simulink model "basic_04_sim"  (R2020a)
settings: Solver=FixedStepAuto  StartTime=0.0  StopTime=0.8  FixedStep=0.001  RelTol=1e-3  EnableMultiTasking=on
values from neighbouring files (symbols this model uses):
  m = size(traj)    [testInput.m]
undefined symbols (not defined in the file or in its folder): a1, a2, a3, d1, d4, fc1, fc2, fc3, fc4, fc5, fc6, fv1, fv2, fv3, fv4, fv5, fv6, Ic111, Ic112, Ic113, Ic122, Ic123, Ic133, Ic211, Ic212, Ic213, Ic222, Ic223, Ic233, Ic311, Ic312, Ic313, Ic322, Ic323, Ic333, Ic411, Ic412, Ic413, Ic422, Ic423, Ic433, Ic511, Ic512, Ic513, Ic522, Ic523, Ic533, Ic611, Ic612, Ic613, Ic622, Ic623, Ic633, m1, m2, m3, m4, m5, m6, mc11 ... (+20)
libraries: sm_lib x56, nesl_utility x31
(part 2 of 2)

== matlab function basic_04_sim/ddq6 ==
  data: u input; y output
function y = fcn(u)  
% if u < 0.5    
%     y = -3.14^3*sin(3.14*u);
% else
%     y = -3.14^3*sin(3.14*(1-u));
% end
% y = 10*sin(u);

q0 = 0;
q1 = pi/6;
% q1 = 0;
acc0 = 0;
acc1 = 0; 
t1 = 0.88;
t0 = 0;
v0 = 0;
v1 = 0;

dq = q1-q0;%初始角度差
dt = t1-t0;%时间差

a0 = q0;
a1 = v0;
a2 = acc0/2;
a3 = (20*dq-(8*v1+12*v0)*dt-(3*acc0-acc1)*dt^2)/(2*dt^3);
a4 = (-30*dq+(14*v1+16*v0)*dt+(3*acc0-2*acc1)*dt^2)/(2*dt^4);
a5 = (12*dq-6*(v1+v0)*dt-(acc0-acc1)*dt^2)/(2*dt^5);

y = 2*a2+6*a3*u+12*a4*u.^2+20*a5*u.^3;%角速度

end

== matlab function basic_04_sim/dq6 ==
  data: u input; y output
function y = fcn(u)  
% if u < 0.5    
%     y = 3.14*3.14*cos(3.14*u);
% else
%     y = -3.14*3.14*cos(3.14*(1-u));
% end

q0 = 0;
q1 = pi/6;
% q1 = 0;
acc0 = 0;
acc1 = 0; 
t1 = 0.88;
t0 = 0;
v0 = 0;
v1 = 0;

dq = q1-q0;%初始角度差
dt = t1-t0;%时间差

a0 = q0;
a1 = v0;
a2 = acc0/2;
a3 = (20*dq-(8*v1+12*v0)*dt-(3*acc0-acc1)*dt^2)/(2*dt^3);
a4 = (-30*dq+(14*v1+16*v0)*dt+(3*acc0-2*acc1)*dt^2)/(2*dt^4);
a5 = (12*dq-6*(v1+v0)*dt-(acc0-acc1)*dt^2)/(2*dt^5);

y = a1+2*a2*u+3*a3*u.^2+4*a4*u.^3+5*a5*u.^4;%角速度
end

== matlab function basic_04_sim/q6 ==
  data: u input; y output
function y = fcn(u)  
% if u < 0.5    
%     y = 3.14*sin(3.14*u);
% else
%     y = 3.14*sin(3.14*(1-u));
% end
q0 = 0;
q1 = pi/6;
% q1 = 0;
acc0 = 0;
acc1 = 0; 
t1 = 0.88;
t0 = 0;
v0 = 0;
v1 = 0;

dq = q1-q0;%初始角度差
dt = t1-t0;%时间差

a0 = q0;
a1 = v0;
a2 = acc0/2;
a3 = (20*dq-(8*v1+12*v0)*dt-(3*acc0-acc1)*dt^2)/(2*dt^3);
a4 = (-30*dq+(14*v1+16*v0)*dt+(3*acc0-2*acc1)*dt^2)/(2*dt^4);
a5 = (12*dq-6*(v1+v0)*dt-(acc0-acc1)*dt^2)/(2*dt^5);

y = a0+a1*u+a2*u.^2+a3*u.^3+a4*u.^4+a5*u.^5;%角度

end

== matlab function basic_04_sim/q1 ==
  data: u input; y output
function y = fcn(u)  
% if u < 0.5    
%     y = 3.14*sin(3.14*u);
% else
%     y = 3.14*sin(3.14*(1-u));
% end
q0 = 0;
q1 = pi/3;
acc0 = 0;
acc1 = 0; 
t1 = 0.88;
t0 = 0;
v0 = 0;
v1 = 0;

dq = q1-q0;%初始角度差
dt = t1-t0;%时间差

a0 = q0;
a1 = v0;
a2 = acc0/2;
a3 = (20*dq-(8*v1+12*v0)*dt-(3*acc0-acc1)*dt^2)/(2*dt^3);
a4 = (-30*dq+(14*v1+16*v0)*dt+(3*acc0-2*acc1)*dt^2)/(2*dt^4);
a5 = (12*dq-6*(v1+v0)*dt-(acc0-acc1)*dt^2)/(2*dt^5);

y = a0+a1*u+a2*u.^2+a3*u.^3+a4*u.^4+a5*u.^5;%角度

end

== matlab function basic_04_sim/ddq1 ==
  data: u input; y output
function y = fcn(u)  
% if u < 0.5    
%     y = -3.14^3*sin(3.14*u);
% else
%     y = -3.14^3*sin(3.14*(1-u));
% end
% y = 10*sin(u);

q0 = 0;
q1 = pi/3;
acc0 = 0;
acc1 = 0; 
t1 = 0.88;
t0 = 0;
v0 = 0;
v1 = 0;

dq = q1-q0;%初始角度差
dt = t1-t0;%时间差

a0 = q0;
a1 = v0;
a2 = acc0/2;
a3 = (20*dq-(8*v1+12*v0)*dt-(3*acc0-acc1)*dt^2)/(2*dt^3);
a4 = (-30*dq+(14*v1+16*v0)*dt+(3*acc0-2*acc1)*dt^2)/(2*dt^4);
a5 = (12*dq-6*(v1+v0)*dt-(acc0-acc1)*dt^2)/(2*dt^5);

y = 2*a2+6*a3*u+12*a4*u.^2+20*a5*u.^3;%角速度

end

== matlab function basic_04_sim/q2 ==
  data: u input; y output
function y = fcn(u)  
% if u < 0.5    
%     y = 3.14*sin(3.14*u);
% else
%     y = 3.14*sin(3.14*(1-u));
% end
q0 = 0;
q1 = pi/6;
% q1 = 0;
acc0 = 0;
acc1 = 0; 
t1 = 0.88;
t0 = 0;
v0 = 0;
v1 = 0;

dq = q1-q0;%初始角度差
dt = t1-t0;%时间差

a0 = q0;
a1 = v0;
a2 = acc0/2;
a3 = (20*dq-(8*v1+12*v0)*dt-(3*acc0-acc1)*dt^2)/(2*dt^3);
a4 = (-30*dq+(14*v1+16*v0)*dt+(3*acc0-2*acc1)*dt^2)/(2*dt^4);
a5 = (12*dq-6*(v1+v0)*dt-(acc0-acc1)*dt^2)/(2*dt^5);

y = a0+a1*u+a2*u.^2+a3*u.^3+a4*u.^4+a5*u.^5;%角度

end

== matlab function basic_04_sim/friction ==
  data: u input; y output; fv input; fc input
function y = fcn(u,fv,fc)
%#codegen

%fv1=100; fc1=80; fv2=150; fc2=100; fv3=100; fc3=50; fv4=80; fc4=80; fv5=50; fc5=30; fv6=30; fc6=10;
% fv1=10; fc1=8; fv2=15; fc2=10; fv3=10; fc3=5; 
% fv4=8; fc4=8; fv5=5; fc5=3; fv6=3; fc6=1;
%fv1=fv(1); fc1=fc(1); fv2=fv(2); fc2=fc(2); fv3=fv(3); fc3=fc(3); fv4=fv(4); fc4=fc(4); fv5=fv(5); fc5=fc(5); fv6=fv(6); fc6=fc(6);
fv1=5; fc1=4; fv2=7; fc2=5; fv3=5; fc3=2.5; 
fv4=4; fc4=4; fv5=2.5; fc5=1.5; fv6=1.5; fc6=1;
% fv1=0; fc1=0; fv2=0; fc2=0; fv3=0; fc3=0; 
% fv4=0; fc4=0; fv5=0; fc5=0; fv6=0; fc6=0;

y=[0;0;0;0;0;0];
y(1)=(fv1*u(1)+fc1*sign(u(1)));
y(2)=(fv2*u(2)+fc2*sign(u(2)));
y(3)=(fv3*u(3)+fc3*sign(u(3)));
y(4)=(fv4*u(4)+fc4*sign(u(4)));
y(5)=(fv5*u(5)+fc5*sign(u(5)));
y(6)=(fv6*u(6)+fc6*sign(u(6)));

end

== matlab function basic_04_sim/dq2 ==
  data: u input; y output
function y = fcn(u)  
% if u < 0.5    
%     y = 3.14*3.14*cos(3.14*u);
% else
%     y = -3.14*3.14*cos(3.14*(1-u));
% end

q0 = 0;
q1 = pi/6;
% q1 = 0;
acc0 = 0;
acc1 = 0; 
t1 = 0.88;
t0 = 0;
v0 = 0;
v1 = 0;

dq = q1-q0;%初始角度差
dt = t1-t0;%时间差

a0 = q0;
a1 = v0;
a2 = acc0/2;
a3 = (20*dq-(8*v1+12*v0)*dt-(3*acc0-acc1)*dt^2)/(2*dt^3);
a4 = (-30*dq+(14*v1+16*v0)*dt+(3*acc0-2*acc1)*dt^2)/(2*dt^4);
a5 = (12*dq-6*(v1+v0)*dt-(acc0-acc1)*dt^2)/(2*dt^5);

y = a1+2*a2*u+3*a3*u.^2+4*a4*u.^3+5*a5*u.^4;%角速度
end

== matlab function basic_04_sim/ddq2 ==
  data: u input; y output
function y = fcn(u)  
% if u < 0.5    
%     y = -3.14^3*sin(3.14*u);
% else
%     y = -3.14^3*sin(3.14*(1-u));
% end
% y = 10*sin(u);

q0 = 0;
q1 = pi/6;
% q1 = 0;
acc0 = 0;
acc1 = 0; 
t1 = 0.88;
t0 = 0;
v0 = 0;
v1 = 0;

dq = q1-q0;%初始角度差
dt = t1-t0;%时间差

a0 = q0;
a1 = v0;
a2 = acc0/2;
a3 = (20*dq-(8*v1+12*v0)*dt-(3*acc0-acc1)*dt^2)/(2*dt^3);
a4 = (-30*dq+(14*v1+16*v0)*dt+(3*acc0-2*acc1)*dt^2)/(2*dt^4);
a5 = (12*dq-6*(v1+v0)*dt-(acc0-acc1)*dt^2)/(2*dt^5);

y = 2*a2+6*a3*u+12*a4*u.^2+20*a5*u.^3;%角速度

end

== matlab function basic_04_sim/ddq3 ==
  data: u input; y output
function y = fcn(u)  

q0 = 0;
q1 = pi/4;
% q1 = 0;
acc0 = 0;
acc1 = 0; 
t1 = 0.88;
t0 = 0;
v0 = 0;
v1 = 0;

dq = q1-q0;%初始角度差
dt = t1-t0;%时间差

a0 = q0;
a1 = v0;
a2 = acc0/2;
a3 = (20*dq-(8*v1+12*v0)*dt-(3*acc0-acc1)*dt^2)/(2*dt^3);
a4 = (-30*dq+(14*v1+16*v0)*dt+(3*acc0-2*acc1)*dt^2)/(2*dt^4);
a5 = (12*dq-6*(v1+v0)*dt-(acc0-acc1)*dt^2)/(2*dt^5);

y = 2*a2+6*a3*u+12*a4*u.^2+20*a5*u.^3;%角速度

end

== matlab function basic_04_sim/dq3 ==
  data: u input; y output
function y = fcn(u)  

q0 = 0;
q1 = pi/4;
% q1 = 0;
acc0 = 0;
acc1 = 0; 
t1 = 0.88;
t0 = 0;
v0 = 0;
v1 = 0;

dq = q1-q0;%初始角度差
dt = t1-t0;%时间差

a0 = q0;
a1 = v0;
a2 = acc0/2;
a3 = (20*dq-(8*v1+12*v0)*dt-(3*acc0-acc1)*dt^2)/(2*dt^3);
a4 = (-30*dq+(14*v1+16*v0)*dt+(3*acc0-2*acc1)*dt^2)/(2*dt^4);
a5 = (12*dq-6*(v1+v0)*dt-(acc0-acc1)*dt^2)/(2*dt^5);

y = a1+2*a2*u+3*a3*u.^2+4*a4*u.^3+5*a5*u.^4;%角速度
end

== matlab function basic_04_sim/q3 ==
  data: u input; y output
function y = fcn(u)  

q0 = 0;
q1 = pi/4;
% q1 = 0;
acc0 = 0;
acc1 = 0; 
t1 = 0.88;
t0 = 0;
v0 = 0;
v1 = 0;

dq = q1-q0;%初始角度差
dt = t1-t0;%时间差

a0 = q0;
a1 = v0;
a2 = acc0/2;
a3 = (20*dq-(8*v1+12*v0)*dt-(3*acc0-acc1)*dt^2)/(2*dt^3);
a4 = (-30*dq+(14*v1+16*v0)*dt+(3*acc0-2*acc1)*dt^2)/(2*dt^4);
a5 = (12*dq-6*(v1+v0)*dt-(acc0-acc1)*dt^2)/(2*dt^5);

y = a0+a1*u+a2*u.^2+a3*u.^3+a4*u.^4+a5*u.^5;%角度

end

== matlab function basic_04_sim/ddq4 ==
  data: u input; y output
function y = fcn(u)  
% if u < 0.5    
%     y = -3.14^3*sin(3.14*u);
% else
%     y = -3.14^3*sin(3.14*(1-u));
% end
% y = 10*sin(u);

q0 = 0;
q1 = pi/5;
% q1 = 0;
acc0 = 0;
acc1 = 0; 
t1 = 0.88;
t0 = 0;
v0 = 0;
v1 = 0;

dq = q1-q0;%初始角度差
dt = t1-t0;%时间差

a0 = q0;
a1 = v0;
a2 = acc0/2;
a3 = (20*dq-(8*v1+12*v0)*dt-(3*acc0-acc1)*dt^2)/(2*dt^3);
a4 = (-30*dq+(14*v1+16*v0)*dt+(3*acc0-2*acc1)*dt^2)/(2*dt^4);
a5 = (12*dq-6*(v1+v0)*dt-(acc0-acc1)*dt^2)/(2*dt^5);

y = 2*a2+6*a3*u+12*a4*u.^2+20*a5*u.^3;%角速度

end

== matlab function basic_04_sim/dq4 ==
  data: u input; y output
function y = fcn(u)  

q0 = 0;
q1 = pi/5;
% q1 = 0;
acc0 = 0;
acc1 = 0; 
t1 = 0.88;
t0 = 0;
v0 = 0;
v1 = 0;

dq = q1-q0;%初始角度差
dt = t1-t0;%时间差

a0 = q0;
a1 = v0;
a2 = acc0/2;
a3 = (20*dq-(8*v1+12*v0)*dt-(3*acc0-acc1)*dt^2)/(2*dt^3);
a4 = (-30*dq+(14*v1+16*v0)*dt+(3*acc0-2*acc1)*dt^2)/(2*dt^4);
a5 = (12*dq-6*(v1+v0)*dt-(acc0-acc1)*dt^2)/(2*dt^5);

y = a1+2*a2*u+3*a3*u.^2+4*a4*u.^3+5*a5*u.^4;%角速度
end

== matlab function basic_04_sim/dq1 ==
  data: u input; y output
function y = fcn(u)  
% if u < 0.5    
%     y = 3.14*3.14*cos(3.14*u);
% else
%     y = -3.14*3.14*cos(3.14*(1-u));
% end

q0 = 0;
q1 = pi/3;
acc0 = 0;
acc1 = 0; 
t1 = 0.88;
t0 = 0;
v0 = 0;
v1 = 0;

dq = q1-q0;%初始角度差
dt = t1-t0;%时间差

a0 = q0;
a1 = v0;
a2 = acc0/2;
a3 = (20*dq-(8*v1+12*v0)*dt-(3*acc0-acc1)*dt^2)/(2*dt^3);
a4 = (-30*dq+(14*v1+16*v0)*dt+(3*acc0-2*acc1)*dt^2)/(2*dt^4);
a5 = (12*dq-6*(v1+v0)*dt-(acc0-acc1)*dt^2)/(2*dt^5);

y = a1+2*a2*u+3*a3*u.^2+4*a4*u.^3+5*a5*u.^4;%角速度
end

== matlab function basic_04_sim/q4 ==
  data: u input; y output
function y = fcn(u)  

q0 = 0;
q1 = pi/5;
% q1 = 0;
acc0 = 0;
acc1 = 0; 
t1 = 0.88;
t0 = 0;
v0 = 0;
v1 = 0;

dq = q1-q0;%初始角度差
dt = t1-t0;%时间差

a0 = q0;
a1 = v0;
a2 = acc0/2;
a3 = (20*dq-(8*v1+12*v0)*dt-(3*acc0-acc1)*dt^2)/(2*dt^3);
a4 = (-30*dq+(14*v1+16*v0)*dt+(3*acc0-2*acc1)*dt^2)/(2*dt^4);
a5 = (12*dq-6*(v1+v0)*dt-(acc0-acc1)*dt^2)/(2*dt^5);

y = a0+a1*u+a2*u.^2+a3*u.^3+a4*u.^4+a5*u.^5;%角度

end
